simulink model "uwb_0"  (R2025a)
settings: Solver=VariableStepAuto  StartTime=0.0  StopTime=5e-08  RelTol=1e-3
undefined symbols (not defined in the file or in its folder): dspblkCoreblockFVToolHelper, gcbh
libraries: dspstat3 x1, commrfcorlib x1, dspfiltersrcs x1, dspsigops x1
settings Model: Creator=IWMAI  LastModifiedBy=IWMAI

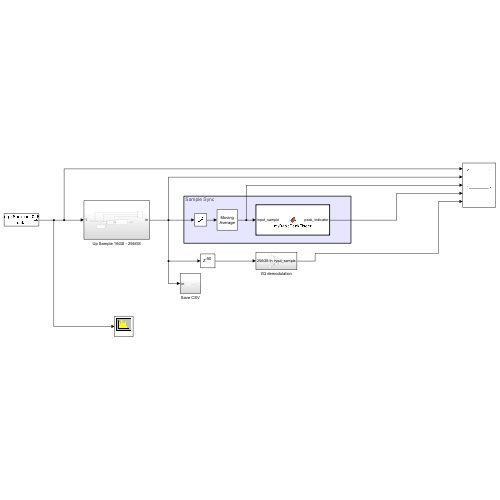
[thumbnail: Simulink's stored preview of the top-level diagram]
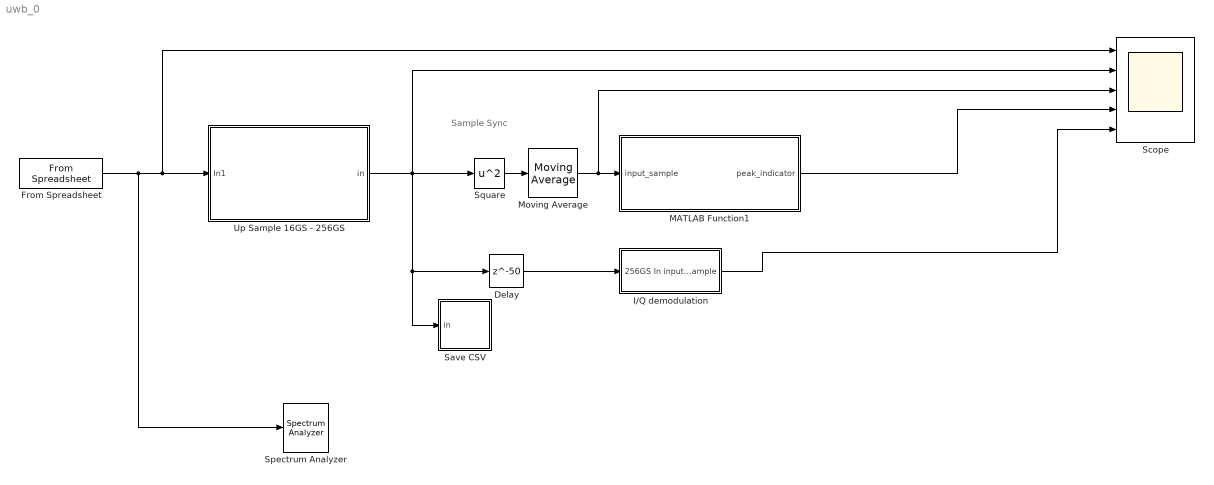
== system uwb_0 ==
  note: Sample Sync
  Delay : Delay  DelayLength=50
  From Spreadsheet : FromSpreadsheet  FileName=C:\Users\IWMAI\University of Toronto\Yu Huang - Summer-2025-sharted\Yongkang\v3_250617\csv\data.csv  SheetName=data  OutDataTypeStr=double  SampleTime=6.25e-11
  I/Q demodulation : Subsystem
  MATLAB Function1 : MATLAB Function  TreatAsAtomicUnit=on
  Moving Average : dspstat3/Moving Average  Method=Sliding window  ForgettingFactorPort=off  SpecifyWindowLength=on  WindowLength=64  OverlapLength=63  AllowArbitraryInputLength=off  ForgettingFactor=0.9  SimulateUsing=Interpreted execution
  Save CSV : Subsystem
  Scope : Scope  NumInputPorts=5
      settings: ActiveDisplayYMinimum=-0.17458315225654225  ActiveDisplayYMaximum=0.15291518939475007
  Spectrum Analyzer : SpectrumAnalyzer  WindowPosition=[624.000000,326.000000,800.000000,500.000000,]  ScopeFrameLocation=window  WindowInvariantSamplesPerUpdate=on  YLimits=[-72.7658 4.4718]
      settings: OpenAtSimulationStart=off
  Square : Math  Operator=square
  Up Sample 16GS - 256GS : Subsystem
  wires:
  From Spreadsheet/1 -> Spectrum Analyzer/1, Up Sample 16GS - 256GS/1(In1), Scope/1
  Square/1 -> Moving Average/1
  Moving Average/1 -> MATLAB Function1/1(input_sample), Scope/3
  MATLAB Function1/1(peak_indicator) -> Scope/4
  Delay/1 -> I/Q demodulation/1(256GS In)
  I/Q demodulation/1(input_sample) -> Scope/5
  Up Sample 16GS - 256GS/1(in) -> Save CSV/1(in), Delay/1, Square/1, Scope/2

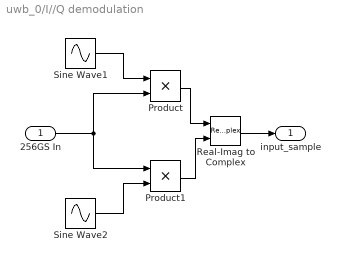
== system uwb_0/I//Q demodulation ==
  256GS In : Inport
  Product : Product
  Product1 : Product
  Real-Imag to Complex : RealImagToComplex
  Sine Wave1 : Sin  Frequency=2 * pi * 3.75e9  Phase=pi/2  SampleTime=0
  Sine Wave2 : Sin  Frequency=2 * pi * 3.75e9  SampleTime=0
  input_sample : Outport
  wires:
  256GS In/1 -> Product/2, Product1/1
  Sine Wave2/1 -> Product1/2
  Sine Wave1/1 -> Product/1
  Product/1 -> Real-Imag to Complex/1
  Product1/1 -> Real-Imag to Complex/2
  Real-Imag to Complex/1 -> input_sample/1

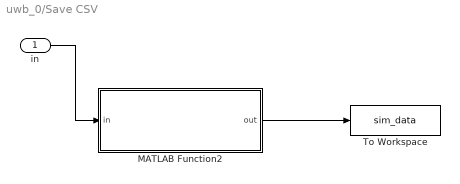
== system uwb_0/Save CSV ==
  in : Inport
  MATLAB Function2 : MATLAB Function  TreatAsAtomicUnit=on
  To Workspace : ToWorkspace  VariableName=sim_data  SaveFormat=Timeseries  SampleTime=-1
  wires:
  MATLAB Function2/1(out) -> To Workspace/1
  in/1 -> MATLAB Function2/1(in)

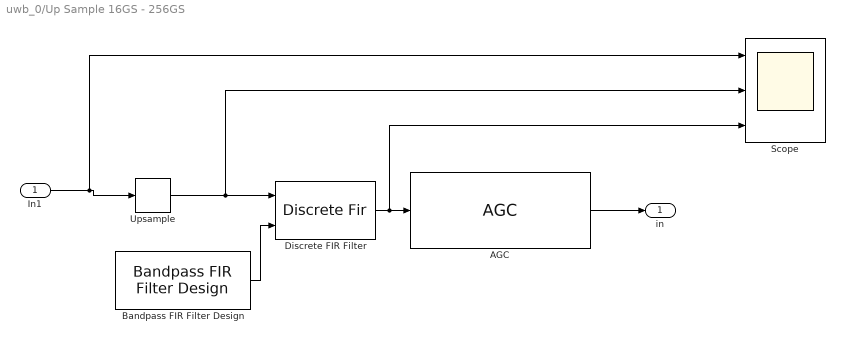
== system uwb_0/Up Sample 16GS - 256GS ==
  In1 : Inport
  AGC : commrfcorlib/AGC  LegacyMode=off  DetectorMethod=Rectifier  LoopMethod=Linear  UpdatePeriod=100  StepSize=0.1  AdaptationStepSize=0.01  DesiredOutputPower=1  AveragingLength=512  MaximumGain=30  MaxPowerGain=60  GainOutputPort=off  InputPowerOutputPort=off  SimulateUsing=Interpreted execution
  Bandpass FIR Filter Design : dspfiltersrcs/Bandpass FIR Filter Design  SmoothParameters=off  SmoothingFactor=0.6  FilterOrderPort=off  FilterOrder=100  MaxOrder=100  CenterFrequencyPort=off  CenterFrequency=1/64  BandwidthPort=off  Bandwidth=0.01  Window=Hann  SidelobeAttenuationPort=off  SidelobeAttenuation=60  KaiserWindowParameterPort=off  KaiserWindowParameter=.5  OutputDataType=double  SampleTime=256e9  SimulateUsing=Interpreted execution
      settings: LibrarySourceBlock=dspfdesign/Bandpass FIR Filter Design
  Discrete FIR Filter : DiscreteFir  LoadFcn=dspblkCoreblockFVToolHelper(gcbh,'load');  CoefSource=Input port
      settings: CopyFcn=dspblkCoreblockFVToolHelper(gcbh,'copy');  DeleteFcn=dspblkCoreblockFVToolHelper(gcbh,'close');  ModelCloseFcn=dspblkCoreblockFVToolHelper(gcbh,'close');  PreSaveFcn=dspblkCoreblockFVToolHelper(gcbh,'presave');  PostSaveFcn=dspblkCoreblockFVToolHelper(gcbh,'postsave');  CloseFcn=dspblkCoreblockFVToolHelper(gcbh,'close');  InputPortMap=u0,u1
  Scope : Scope  NumInputPorts=3
      settings: ActiveDisplayYMinimum=-0.1766463393208148  ActiveDisplayYMaximum=0.16150855826432609
  Upsample : dspsigops/Upsample  FactorSource=Dialog parameter  N=16  Nmax=16  phase=0  RateOptions=Allow multirate processing  ic=0  mode=Unused parameter value
      settings: LibrarySourceBlock=dsphdlsupportsigops/Upsample
  in : Outport
  wires:
  Upsample/1 -> Scope/2, Discrete FIR Filter/1
  Discrete FIR Filter/1 -> Scope/3, AGC/1
  AGC/1 -> in/1
  Bandpass FIR Filter Design/1 -> Discrete FIR Filter/2
  In1/1 -> Scope/1, Upsample/1

== matlab function uwb_0/Save CSV/MATLAB Function2 ==
  data: in input; out output
function out = save_csv(in)
%#codegen
% This function processes one sample at a time.
% To store data across simulation steps, you need to use persistent variables.

persistent data_buffer;
persistent index_counter;

if isempty(data_buffer)
    % Initialize buffer and counter when simulation starts or resets
    data_buffer = zeros(0, 2); % Column 1 for index, Column 2 for data
    index_counter = 0;
end

% Increment index and store current sample
index_counter = index_counter + 1;
data_buffer = [data_buffer; index_counter, in];

% Output the current sample (or anything else you need downstream)
out = in;

% You can add logic here to write to CSV periodically,
% but it's generally better to do it after simulation.
% For this method, we'll let 'To Workspace' handle saving.

% At the end of simulation, the persistent variables will be cleared unless
% you explicitly save them or access them from the base workspace.
% For 'To Workspace' method, it's about the *output* of this block.
end

== matlab function uwb_0/MATLAB Function1 ==
  data: input_sample input; peak_indicator output
function peak_indicator = myBasicPeakFinder(input_sample)
% myBasicPeakFinder: A basic peak detector with min_height, min_distance,
% and a fixed output delay.
%
% input_sample: The current input sample (scalar).
% peak_indicator: Output is 1 if a peak was detected 'OUTPUT_DELAY_C' samples ago,
%                 0 otherwise.

% --- 1. Persistent Variables Declaration and Initialization ---
% These variables maintain their state across function calls.
persistent data_buffer;       % Stores historical input samples (circular buffer)
persistent output_buffer;     % Stores peak detection results for delayed output
persistent head_idx;          % Pointer to the head (oldest element) of data_buffer
persistent tail_idx;          % Pointer to the tail (newest element) of data_buffer
persistent current_abs_idx;   % Absolute index of the current input sample in the stream
persistent last_peak_abs_idx; % Absolute index of the last confirmed peak

% --- 2. Tunable Parameters ---
% Adjust these values based on your signal and requirements.
% Use CONSTANT_VALUE type for these parameters in the MATLAB Function block properties
% if you want them fixed. If you want to change them during simulation,
% you can expose them as input ports to the block.

BUFFER_LEN = 200;           % Input data buffer length. Must be > (MIN_DISTANCE + OUTPUT_DELAY_C).
                            % Ensure it's long enough to contain data needed for peak checking.
OUTPUT_DELAY_C = 50;        % Number of samples to delay the peak indicator output.
                            % When a peak occurs, the 'high' signal appears after this delay.
MIN_HEIGHT = 5e-3;          % Minimum amplitude for a point to be considered a peak.
MIN_DISTANCE = 400;          % Minimum number of samples between two consecutive peaks.

% --- 3. Initialization Logic (executed once at the start of simulation) ---
if isempty(data_buffer)
    data_buffer = zeros(1, BUFFER_LEN);
    output_buffer = zeros(1, OUTPUT_DELAY_C);
    head_idx = 1;
    tail_idx = 0; % Will be incremented to 1 on first sample
    current_abs_idx = 0; % Global sample counter
    last_peak_abs_idx = -inf; % Initialize to negative infinity to allow first peak
end

% --- 4. Update Input Data Buffer (Circular Buffer Logic) ---
current_abs_idx = current_abs_idx + 1; % Increment global sample counter

tail_idx = tail_idx + 1;
if tail_idx > BUFFER_LEN
    tail_idx = 1; % Wrap around
end
data_buffer(tail_idx) = input_sample; % Store new sample

% --- 5. Cold Start / Buffer Fill-up Handling ---
% If the buffer is not yet full, or not enough data for the delay, output low.
% And return early.
if current_abs_idx < BUFFER_LEN % Ensure buffer is fully populated once
    peak_indicator = 0;
    % For output buffer, we also need to fill it with zeros during cold start
    % This ensures the delayed output is correctly initialized.
    output_buffer = [output_buffer(2:end), 0]; % Shift and add a zero
    return;
end

% --- 6. Determine Analysis Point in Buffer ---
% The point we are analyzing is 'OUTPUT_DELAY_C' samples in the past from the current 'tail_idx'.
% This corresponds to the input sample 'current_abs_idx - OUTPUT_DELAY_C'.
analysis_idx_in_buffer = tail_idx - OUTPUT_DELAY_C;
if analysis_idx_in_buffer <= 0
    analysis_idx_in_buffer = analysis_idx_in_buffer + BUFFER_LEN; % Wrap around for circular buffer
end

% Get surrounding indices for local maxima check
prev_idx = analysis_idx_in_buffer - 1;
if prev_idx <= 0
    prev_idx = prev_idx + BUFFER_LEN; % Wrap around
end
next_idx = analysis_idx_in_buffer + 1;
if next_idx > BUFFER_LEN
    next_idx = next_idx - BUFFER_LEN; % Wrap around
end

% Get actual sample values
current_sample_val = data_buffer(analysis_idx_in_buffer);
prev_sample_val = data_buffer(prev_idx);
next_sample_val = data_buffer(next_idx);

% --- 7. Peak Detection Logic (for the analysis_idx_in_buffer point) ---
is_peak_at_analysis_point = false;

% Check min_height
if current_sample_val >= MIN_HEIGHT
    % Check if it's a local maximum (greater than its immediate neighbors)
    % Using > for strict local maxima, could use >= if plateaus are allowed
    if (current_sample_val > prev_sample_val) && (current_sample_val > next_sample_val)
        
        % Get absolute index of the point being analyzed
        abs_idx_of_analysis_point = current_abs_idx - OUTPUT_DELAY_C;

        % Check min_distance
        if (abs_idx_of_analysis_point - last_peak_abs_idx) >= MIN_DISTANCE
            is_peak_at_analysis_point = true;
            last_peak_abs_idx = abs_idx_of_analysis_point; % Update last detected peak's absolute index
        end
    end
end

% --- 8. Update Output Buffer and Get Current Output ---
% The decision for 'is_peak_at_analysis_point' is for a point 'OUTPUT_DELAY_C' samples in the past.
% This decision is now moved into the output_buffer's 'future'.
output_buffer = [output_buffer(2:end), is_peak_at_analysis_point];

% The actual output for the current function call is the oldest element in output_buffer.
peak_indicator = output_buffer(1);

end
